simulink model "BD_PAR_SS"  (Simulink 10.3)
settings: Solver=ode1  StartTime=0.0  StopTime=max(cyc_mph(:,1))  FixedStep=1  MaxStep=1  RelTol=1e-3  AbsTol=1e-3
undefined symbols (not defined in the file): acc_elec_eff, acc_elec_pwr, acc_mech_eff, amb_tmp, cs_charge_deplete_bool, cs_electric_decel_spd, cs_electric_launch_spd_hi, cs_electric_launch_spd_lo, cs_hi_soc, cs_lo_soc, cs_off_trq_frac, cyc_avg_time, cyc_cargo_mass, cyc_elevation_init, cyc_filter_bool, cyc_grade, cyc_mph, ess_module_num, ess_on, ess_voc, ex_calc, ex_cat_co_frac, ex_cat_ext_cp, ex_cat_ext_emisv, ex_cat_ext_init_tmp, ex_cat_ext_mass, ex_cat_ext_sarea, ex_cat_hc_frac, ex_cat_i2p_th_cond, ex_cat_i2x_emisv, ex_cat_i2x_th_cond, ex_cat_int_cp, ex_cat_int_init_tmp, ex_cat_int_mass, ex_cat_int_sarea, ex_cat_lim, ex_cat_m2i_th_cond, ex_cat_m2i_tmp, ex_cat_m2p_emisv, ex_cat_mon_cp, ex_cat_mon_init_tmp, ex_cat_mon_mass, ex_cat_mon_sarea, ex_cat_monf_sarea, ex_cat_moni_sarea, ex_cat_nox_frac, ex_cat_p2x_th_cond, ex_cat_pcm_ecp, ex_cat_pcm_mass, ex_cat_pcm_tmp, ex_cat_pipe_cp, ex_cat_pipe_emisv, ex_cat_pipe_init_tmp, ex_cat_pipe_mass, ex_cat_pipe_sarea, ex_cat_pm_frac, ex_cat_tmp_range, ex_gas_cp, ex_manif_cp, ex_manif_emisv ... (+73)
libraries: lib_controls x6, lib_vehicle x3, lib_accessory x2, lib_interactive x1, lib_energy_storage x1, lib_fuel_converter x1
(part 2 of 6)

== system BD_PAR_SS/mechanical accessory loads <acc> ==
  note: from <fc>
  note: from <fc>
  note: torque req
  note: speed req
  note: aux spd req
  note: torque achieved
  note: speed achieved
  note: aux spd achieved
  note: from <fc>
  note: In order to load the engine,
      | the engine must be on and
      | the shaft speed must
      | be greater than zero (fc_spd_est is assumed
      | to bound itself to max fc speed and idle speed)
      |
      | The basic assumption is that the aux. loads
      | will not change the requested engine speed--
      | only the torque
  note: "kill switch" for accessory loads
  In1 : Inport
  In2 : Inport  Port=2
  Constant : Constant  Value=eps
  Demux : Demux  Outputs=2
      settings: DisplayOption=none
  Demux1 : Demux  Outputs=2
      settings: DisplayOption=none
  Logical Operator : Logic
  Mechanical Accessory Loads v2 <acc> : Subsystem  mask{load_on=not(ess_on)*1, acc_max_spd=inf, acc_min_spd=vc_idle_spd*vc_idle_bool+eps, ic_mech_trq=0, ic_mech_pwr=0}
      mask prompts: load_on "Electrical Load Status: 1 on; 0 off"; acc_max_spd "maximum shaft speed for aux. (rad/s)"; acc_min_spd "minimum shaft speed for aux. (rad/s)"; ic_mech_trq "Initial Mechanical Torque of the Accessory Loads (Nm)"; ic_mech_pwr "Initial Mechanical Auxiliary Load Power (W)"
      mask Display: image(imread('bdi_acc_pic.bmp'))
  Mux : Mux  Inputs=3
  Mux1 : Mux  Inputs=3
  Relational Operator : RelationalOperator  Operator=>  RndMeth=Nearest  InputSameDT=on
  Out1 : Outport
  Out2 : Outport  Port=2
  wires:
  [signal_one] -> Mechanical Accessory Loads v2 <acc>/1("requested shaft T and w, out to the driveline  (Nm ; rad/s; rad/s)")
  Mechanical Accessory Loads v2 <acc>/1("requested shaft and belt T and w, in from the prime mover (Nm ; rad/s)") -> Out1/1
  Mechanical Accessory Loads v2 <acc>/2("achieved shaft T and w, out to the driveline (Nm ; rad/s)") -> Out2/1
  [signal_two] -> Mechanical Accessory Loads v2 <acc>/2("achieved shaft and belt T and w, in from the prime mover (Nm ; rad/s)")
  Mux/1 -> [signal_one]
  In1/1 -> Demux/1
  Demux/1 -> Mux/1
  Demux/2 -> Mux/2
  [fc_spd_est] -> Mux/3
  Mux1/1 -> [signal_two]
  In2/1 -> Demux1/1
  Demux1/1 -> Mux1/1
  Demux1/2 -> Mux1/2
  [fc_spd_est] -> Mux1/3
  [engine_on] -> Logical Operator/1
  Logical Operator/1 -> [acc_on]
  [acc_on] -> Mechanical Accessory Loads v2 <acc>/3(accessory on/off)
  [fc_spd_est] -> Relational Operator/1
  Constant/1 -> Relational Operator/2
  Relational Operator/1 -> Logical Operator/2

== system BD_PAR_SS/motor/ controller <mc> par ==
  "torque and speed  req'd at rotor (Nm), (rad/s)" : Inport
  available motor input power (W) : Inport  Port=2
  Block NOTES : Subsystem
      mask Display: disp('Block\nNOTES')
  Constant : Constant  Value=mc_eff_scale
  Demux : Demux  Outputs=2
  Fcn : Fcn  Expr=u[3]-u[1]*u[2]
  Mux2 : Mux  Inputs=2
  Mux3 : Mux  Inputs=3
  N-m drive torque per W input : Subsystem
  Product : Product  SaturateOnIntegerOverflow=on
  Product1 : Product  Inputs=*/  SaturateOnIntegerOverflow=on
  Saturation : Saturate  UpperLimit=max(mc_map_spd)*mc_spd_scale  LowerLimit=0
  Sum : Sum  SaturateOnIntegerOverflow=on
  Sum1 : Sum  Inputs=-+  SaturateOnIntegerOverflow=on
  Switch : Switch  SaturateOnIntegerOverflow=on  InputSameDT=on
  To WS1 : ToWorkspace  VariableName=mc_pwr_loss
      settings: MaxDataPoints=50000
  To WS2 : ToWorkspace  VariableName=mc_tmp
      settings: MaxDataPoints=50000
  To WS4 : ToWorkspace  VariableName=mc_clt_th_pwr
      settings: MaxDataPoints=50000
  To Workspace10 : ToWorkspace  VariableName=mc_ni_trq_out_a  SampleTime=-1
  To Workspace4 : ToWorkspace  VariableName=mc_trq_out_r  SampleTime=-1
  To Workspace5 : ToWorkspace  VariableName=mc_spd_out_r  SampleTime=-1
  To Workspace8 : ToWorkspace  VariableName=mc_pwr_in_a  SampleTime=-1
  To Workspace9 : ToWorkspace  VariableName=mc_pwr_in_r  SampleTime=-1
  do ex calcs? : Constant  Value=mc_th_calc
  documentation10 : Subsystem
      settings: OpenFcn=web(['file:\\\' which('motor_controller.htm')]);
      mask Display: image(imread('doc_man.jpg'))
  effect of inertia (Nm) : Subsystem
  enforce torque limit : Subsystem
  mc tmp : Subsystem  TreatAsAtomicUnit=on
  motor controller logic interface : Subsystem
  motor speed estimator : Subsystem
  motor/controller input power map (W) : Lookup2D  RowIndex=mc_map_spd*mc_spd_scale  ColumnIndex=mc_map_trq*mc_trq_scale  Table=mc_inpwr_map*mc_spd_scale*mc_trq_scale  SaturateOnIntegerOverflow=on  InputSameDT=on
  rotor drive torque available (Nm) : Subsystem
  req'd motor input power (W) : Outport  InitialOutput=0
  "drive torque and speed avail. at rotor (Nm), (rad/s)" : Outport  Port=2  InitialOutput=0
  tag scope: mc_spd_out_a=global, mc_trq_out_a=global
  wires:
  motor/controller input power map (W)/1 -> Product/1, Switch/2, Product1/1
  Product/1 -> Switch/3
  Product1/1 -> Switch/1
  Switch/1 -> N-m drive torque per W input/1(req'd input power (W)), motor controller logic interface/2(P_mc_in_1lim)
  Constant/1 -> Product/2, Product1/2
  motor speed estimator/1(Out1) -> motor/controller input power map (W)/1, enforce torque limit/2(limited motor speed (rad/s))
  Saturation/1 -> effect of inertia (Nm)/1(mc_spd_out_a), motor speed estimator/1(mc_spd_out_a), Mux3/2, Mux2/2, [mc_spd_out_a]
  Sum1/1 -> Mux3/1, Mux2/1, [mc_trq_out_a]
  N-m drive torque per W input/1(Nm per W) -> rotor drive torque available (Nm)/1(torque per unit input power (N-m/W))
  Sum/1 -> enforce torque limit/1(req'd motor torque (Nm))
  effect of inertia (Nm)/1(out_1) -> Sum/2, Sum1/1
  enforce torque limit/1(limited motor torque (Nm)) -> N-m drive torque per W input/2(req'd rotor drive torque (Nm)), motor/controller input power map (W)/2
  motor controller logic interface/1(P_mc_in_r) -> To Workspace9/1, req'd motor input power (W)/1
  Mux2/1 -> "drive torque and speed avail. at rotor (Nm), (rad/s)"/1
  Mux3/1 -> Fcn/1
  Fcn/1 -> To WS1/1, mc tmp/1(Qmc_gen)
  do ex calcs?/1 -> mc tmp/Enable
  mc tmp/1(Tmc) -> To WS2/1
  mc tmp/2(Qmc_clt) -> To WS4/1
  [v_prev] -> mc tmp/2(veh spd)
  [key_on] -> mc tmp/3(key ON?)
  Demux/2 -> Saturation/1, To Workspace5/1, motor controller logic interface/1(w_mc_out_r)
  available motor input power (W)/1 -> Mux3/3, To Workspace8/1, rotor drive torque available (Nm)/2(available input power (W))
  Demux/1 -> Sum/1, To Workspace4/1
  "torque and speed  req'd at rotor (Nm), (rad/s)"/1 -> Demux/1
  rotor drive torque available (Nm)/1(rotor drive torque available) -> Sum1/2, To Workspace10/1

== system BD_PAR_SS/par <cs> config ==
  "trq and spd req'd into clutch (N*m, rad/s)" : Inport
  electric assist control strategy <cs> : lib_controls/electric assist control strategy <cs>  SystemSampleTime=-1  VariantActivationTime=update diagram  Latency=0  AutoFrameSizeCalculation=off
  "trq and spd req'd from engine (N*m, rad/s)" : Outport
  wires:
  "trq and spd req'd into clutch (N*m, rad/s)"/1 -> electric assist control strategy <cs>/1
  electric assist control strategy <cs>/1 -> "trq and spd req'd from engine (N*m, rad/s)"/1

== system BD_PAR_SS/power bus <pb> ==
  req'd power output (W) : Inport
  power available from generator (W) : Inport  Port=2
  power available from energy storage (W) : Inport  Port=3
  Abs : Abs  SaturateOnIntegerOverflow=on
  Abs1 : Abs  SaturateOnIntegerOverflow=on
  Block NOTES : Subsystem
      mask Display: disp('Block\nNOTES')
  Constant : Constant  Value=1e-9
  Constant1 : Constant  Value=1e-11
  Constant2 : Constant  Value=0
  Constant7 : Constant  Value=ess_on
  Constant8 : Constant  Value=0
  Relational Operator : RelationalOperator  Operator=<=  RndMeth=Nearest  InputSameDT=on
  Relational Operator1 : RelationalOperator  Operator=<=  RndMeth=Nearest  InputSameDT=on
  Sum1 : Sum  Inputs=+-  SaturateOnIntegerOverflow=on
  Sum2 : Sum  SaturateOnIntegerOverflow=on
  Switch : Switch  Threshold=eps  SaturateOnIntegerOverflow=on  InputSameDT=on
  Switch1 : Switch  Threshold=eps  SaturateOnIntegerOverflow=on  InputSameDT=on
  To Workspace8 : ToWorkspace  VariableName=pb_pwr_out_a  SampleTime=-1
  To Workspace9 : ToWorkspace  VariableName=pb_pwr_out_r  SampleTime=-1
  not(and(u1,u2)) : Logic  Operator=NAND
  power req'd from generator (W) : Outport
  power req'd from energy storage (W) : Outport  Port=2
  output power  available at bus : Outport  Port=3
  wires:
  power available from energy storage (W)/1 -> Sum2/2
  Constant8/1 -> Switch1/3
  Constant7/1 -> Switch1/2
  Switch1/1 -> power req'd from energy storage (W)/1
  Sum1/1 -> Switch1/1
  Constant/1 -> Relational Operator/2
  Abs/1 -> Relational Operator/1
  Sum2/1 -> Switch/1, Abs/1
  Switch/1 -> output power  available at bus/1, To Workspace8/1
  Constant1/1 -> Relational Operator1/2
  Abs1/1 -> Relational Operator1/1
  Relational Operator1/1 -> not(and(u1,u2))/2
  not(and(u1,u2))/1 -> Switch/2
  Constant2/1 -> Switch/3
  Relational Operator/1 -> not(and(u1,u2))/1
  power available from generator (W)/1 -> Sum1/2, Sum2/1
  req'd power output (W)/1 -> power req'd from generator (W)/1, Sum1/1, To Workspace9/1, Abs1/1

== system BD_PAR_SS/torque coupler <tc> ==
  "torque and speed req'd at output side of torque coupler (Nm), (rad/s)" : Inport
  "torque and speed avail. at main input (Nm), (rad/s)" : Inport  Port=2
  "torque and speed avail. at motor input to tc (Nm), (rad/s)" : Inport  Port=3
  Block NOTES : Subsystem
      mask Display: disp('Block\nNOTES')
  Demux : Demux  Outputs=2
  Demux1 : Demux  Outputs=2
  Demux2 : Demux  Outputs=2
  MinMax : MinMax  Inputs=2
  MinMax1 : MinMax  Inputs=2
  Mux : Mux  Inputs=2
  Mux1 : Mux  Inputs=2
  Mux2 : Mux  Inputs=2
  Product : Product  Inputs=1  SaturateOnIntegerOverflow=on
  Product1 : Product  Inputs=1  SaturateOnIntegerOverflow=on
  To Workspace2 : ToWorkspace  VariableName=tc_trq_out_r  SampleTime=-1
  To Workspace3 : ToWorkspace  VariableName=tc_spd_out_r  SampleTime=-1
  To Workspace4 : ToWorkspace  VariableName=tc_trq_out_a  SampleTime=-1
  To Workspace5 : ToWorkspace  VariableName=tc_spd_out_a  SampleTime=-1
  To Workspace6 : ToWorkspace  VariableName=tc_pwr_in_a  SampleTime=-1
  effect of motor torque at output of tc (Nm) : Gain  Gain=tc_mc_to_fc_ratio  SaturateOnIntegerOverflow=on
  help : Subsystem
      settings: OpenFcn=web(['file:\\\' which('torque_coupler.htm')]);
      mask Display: image(imread('doc_man.jpg'))
  loss (Nm) : Subsystem
  speed of output gear corresponding to motor spd (rad/s) : Gain  Gain=1/tc_mc_to_fc_ratio  SaturateOnIntegerOverflow=on
  speed req'd of motor (rad/s) : Gain  Gain=tc_mc_to_fc_ratio  SaturateOnIntegerOverflow=on
  "sum " : Sum  SaturateOnIntegerOverflow=on
  torque avail. at output side of tc (Nm) : Sum  Inputs=-++  SaturateOnIntegerOverflow=on
  total torque req'd at output gear (Nm) : Sum  SaturateOnIntegerOverflow=on
  total torque req'd of motor (Nm) : Gain  Gain=1/tc_mc_to_fc_ratio  SaturateOnIntegerOverflow=on
  unmet torque request (Nm) : Sum  Inputs=+-  SaturateOnIntegerOverflow=on
  "torque and speed req'd at main input to torque coupler (Nm), (rad/s)" : Outport  InitialOutput=0
  "torque and speed req'd at motor input to torque coupler (Nm), (rad/s)" : Outport  Port=2  InitialOutput=0
  "torque and speed avail. at output side of torque coupler (Nm), (rad/s)" : Outport  Port=3  InitialOutput=0
  wires:
  Product1/1 -> "sum "/2
  "torque and speed avail. at motor input to tc (Nm), (rad/s)"/1 -> Product1/1, Demux2/1
  "torque and speed avail. at main input (Nm), (rad/s)"/1 -> Product/1, Demux1/1
  Product/1 -> "sum "/1
  "sum "/1 -> To Workspace6/1
  Mux/1 -> "torque and speed req'd at main input to torque coupler (Nm), (rad/s)"/1
  "torque and speed req'd at output side of torque coupler (Nm), (rad/s)"/1 -> Demux/1
  Demux/2 -> loss (Nm)/1(tc output speed (rad/s)), Mux/2, MinMax/1, To Workspace3/1
  total torque req'd at output gear (Nm)/1 -> Mux/1, unmet torque request (Nm)/1
  unmet torque request (Nm)/1 -> total torque req'd of motor (Nm)/1
  Demux1/2 -> MinMax/2
  Mux1/1 -> "torque and speed req'd at motor input to torque coupler (Nm), (rad/s)"/1
  total torque req'd of motor (Nm)/1 -> Mux1/1
  speed req'd of motor (rad/s)/1 -> Mux1/2
  loss (Nm)/1(drag torque (Nm)) -> total torque req'd at output gear (Nm)/2, torque avail. at output side of tc (Nm)/1
  Demux1/1 -> unmet torque request (Nm)/2, torque avail. at output side of tc (Nm)/2
  Demux2/1 -> effect of motor torque at output of tc (Nm)/1
  effect of motor torque at output of tc (Nm)/1 -> torque avail. at output side of tc (Nm)/3
  Mux2/1 -> "torque and speed avail. at output side of torque coupler (Nm), (rad/s)"/1
  Demux2/2 -> speed of output gear corresponding to motor spd (rad/s)/1
  speed of output gear corresponding to motor spd (rad/s)/1 -> MinMax1/2
  MinMax/1 -> speed req'd of motor (rad/s)/1, MinMax1/1
  Demux/1 -> total torque req'd at output gear (Nm)/1, To Workspace2/1
  torque avail. at output side of tc (Nm)/1 -> Mux2/1, To Workspace4/1
  MinMax1/1 -> Mux2/2, To Workspace5/1

== system BD_PAR_SS/vehicle <veh> ==
  vehicle speed req'd at end of time step (m/s) : Inport
  tractive force and linear speed achievable (N) : Inport  Port=2
  "(m/s) -> (mph)1" : Gain  Gain=2.23713646532438  SaturateOnIntegerOverflow=on
  Block NOTES : Subsystem
      mask Display: disp('Block\nNOTES')
  Demux1 : Demux  Outputs=2
  Gain : Gain  Gain=0.5  SaturateOnIntegerOverflow=on
  Memory : Memory  InitialCondition=cyc_mph(1,2)*.447
  Mux : Mux  Inputs=2
  Rolling Resistance Force (N) : ToWorkspace  VariableName=Fr  SampleTime=-1
  Sum : Sum  SaturateOnIntegerOverflow=on
  Sum1 : Sum  Inputs=++++  SaturateOnIntegerOverflow=on
  To Workspace2 : ToWorkspace  VariableName=veh_force_r  SampleTime=-1
  To Workspace3 : ToWorkspace  VariableName=veh_spd_r  SampleTime=-1
  To Workspace4 : ToWorkspace  VariableName=veh_force_a  SampleTime=-1
  To Workspace5 : ToWorkspace  VariableName=veh_spd_a  SampleTime=-1
  force req'd to accelerate (N) : Subsystem
  force req'd to ascend (N) : Subsystem
  force req'd to overcome aerodynamic drag (N) : Subsystem
  help : Subsystem
      settings: OpenFcn=web(['file:\\\' which('vehicle.htm')]);
      mask Display: image(imread('doc_man.jpg'))
  record achieved force outputs : Subsystem
  rolling resistance force : Subsystem  BlockChoice=force req'd to overcome rolling resistance (N)
      settings: AttributesFormatString=%<BlockChoice>  TemplateBlock=lib_vehicle/Submodels/rolling resistance force  MemberBlocks=force req'd to overcome rolling resistance (N),force req'd to overcome rolling resistance (N) j2452
  vehicle speed : Subsystem  BlockChoice=vehicle speed (m/s)
      settings: AttributesFormatString=%<BlockChoice>  TemplateBlock=lib_vehicle/Submodels/vehicle speed  MemberBlocks=vehicle speed (m/s),vehicle speed (m/s) j2452
  "tractive force and speed required of tire and wheel (N), (m/s)" : Outport  InitialOutput=0
  tag scope: mpha=global, v_prev=global
  wires:
  vehicle speed/1(vehicle speed achievable at end of time step (m/s)) -> record achieved force outputs/2(spd), "(m/s) -> (mph)1"/1, Memory/1
  tractive force and linear speed achievable (N)/1 -> vehicle speed/2("available tractive force and linear speed (N), (m/s)"), Demux1/1
  Gain/1 -> rolling resistance force/1(average vehicle speed over time step (m/s)), force req'd to overcome aerodynamic drag (N)/1(average vehicle speed over time step (m/s)), Mux/2, To Workspace3/1, force req'd to ascend (N)/1(average vehicle speed over time step (m/s))
  Sum/1 -> Gain/1
  vehicle speed req'd at end of time step (m/s)/1 -> force req'd to accelerate (N)/1(v(m/s)), Sum/1
  Mux/1 -> "tractive force and speed required of tire and wheel (N), (m/s)"/1
  Sum1/1 -> Mux/1, To Workspace2/1
  Demux1/1 -> To Workspace4/1
  Demux1/2 -> To Workspace5/1
  force req'd to overcome aerodynamic drag (N)/1(D aero(N)) -> Sum1/3
  force req'd to accelerate (N)/1((N)) -> Sum1/4
  Memory/1 -> record achieved force outputs/1(spd_prev), [v_prev], vehicle speed/1(vehicle speed at beginning of time step (m/s)), force req'd to accelerate (N)/2(v prev), Sum/2
  "(m/s) -> (mph)1"/1 -> [mpha]
  force req'd to ascend (N)/1((N)) -> Sum1/2
  rolling resistance force/1(Fr (N)) -> Rolling Resistance Force (N)/1, Sum1/1

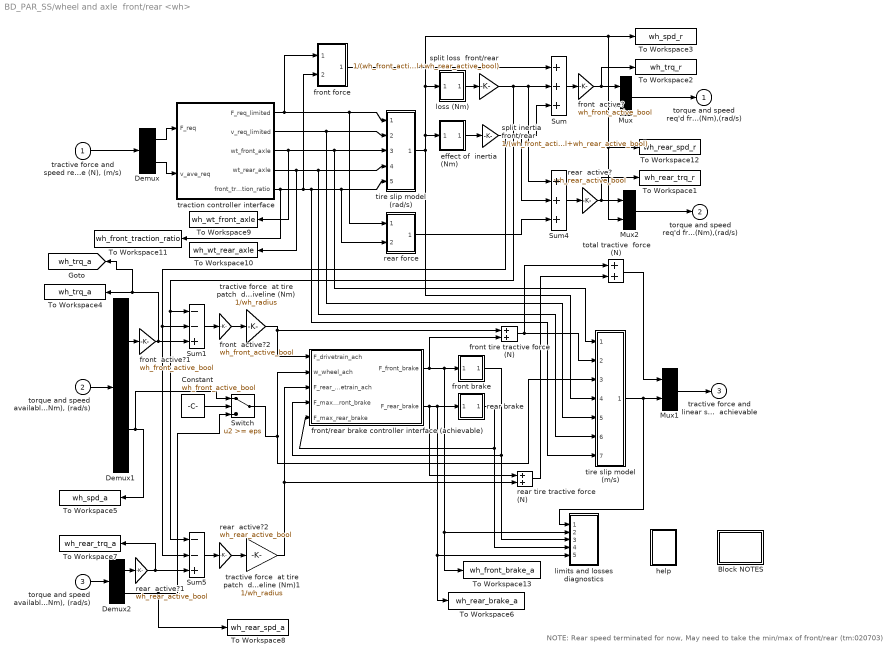
== system BD_PAR_SS/wheel and axle  front/rear <wh> ==
  note: NOTE: Rear speed terminated for now, May need to take the min/max of front/rear (tm:020703)
  "tractive force and speed req'd of tire/road interface (N), (m/s)" : Inport
  "torque and speed available from drivetrain into front axle (Nm), (rad/s)" : Inport  Port=2
  "torque and speed available from drivetrain into rear axle (Nm), (rad/s)" : Inport  Port=3
  Block NOTES : Subsystem
      mask Display: disp('Block\nNOTES')
  Constant : Constant  Value=wh_front_active_bool
  Demux : Demux  Outputs=2
  Demux1 : Demux  Outputs=2
  Demux2 : Demux  Outputs=2
  Mux : Mux  Inputs=2
  Mux1 : Mux  Inputs=2
  Mux2 : Mux  Inputs=2
  Sum : Sum  Inputs=+++  SaturateOnIntegerOverflow=on
  Sum1 : Sum  Inputs=--+  SaturateOnIntegerOverflow=on
  Sum4 : Sum  Inputs=+++  SaturateOnIntegerOverflow=on
  Sum5 : Sum  Inputs=--+  SaturateOnIntegerOverflow=on
  Switch : Switch  Threshold=eps  SaturateOnIntegerOverflow=on  InputSameDT=on
  To Workspace1 : ToWorkspace  VariableName=wh_rear_trq_r  SampleTime=-1
  To Workspace10 : ToWorkspace  VariableName=wh_wt_rear_axle  SampleTime=-1
  To Workspace11 : ToWorkspace  VariableName=wh_front_traction_ratio  SampleTime=-1
  To Workspace12 : ToWorkspace  VariableName=wh_rear_spd_r  SampleTime=-1
  To Workspace13 : ToWorkspace  VariableName=wh_front_brake_a  SampleTime=-1
  To Workspace2 : ToWorkspace  VariableName=wh_trq_r  SampleTime=-1
  To Workspace3 : ToWorkspace  VariableName=wh_spd_r  SampleTime=-1
  To Workspace4 : ToWorkspace  VariableName=wh_trq_a  SampleTime=-1
  To Workspace5 : ToWorkspace  VariableName=wh_spd_a  SampleTime=-1
  To Workspace6 : ToWorkspace  VariableName=wh_rear_brake_a  SampleTime=-1
  To Workspace7 : ToWorkspace  VariableName=wh_rear_trq_a  SampleTime=-1
  To Workspace8 : ToWorkspace  VariableName=wh_rear_spd_a  SampleTime=-1
  To Workspace9 : ToWorkspace  VariableName=wh_wt_front_axle  SampleTime=-1
  effect of  inertia (Nm) : Subsystem
  front  active? : Gain  Gain=wh_front_active_bool  SaturateOnIntegerOverflow=on
  front  active?1 : Gain  Gain=wh_front_active_bool  SaturateOnIntegerOverflow=on
  front  active?2 : Gain  Gain=wh_front_active_bool  SaturateOnIntegerOverflow=on
  front brake : Subsystem
  front force : Subsystem
  front tire tractive force (N) : Sum  SaturateOnIntegerOverflow=on
  front/rear brake controller interface (achievable) : Subsystem
  help : Subsystem
      settings: OpenFcn=web(['file:\\\' which('advisor_doc.htm')]);
      mask Display: image(imread('doc_man.jpg'))
  limits and losses diagnostics : Subsystem
  loss (Nm) : Subsystem
  rear  active? : Gain  Gain=wh_rear_active_bool  SaturateOnIntegerOverflow=on
  rear  active?1 : Gain  Gain=wh_rear_active_bool  SaturateOnIntegerOverflow=on
  rear  active?2 : Gain  Gain=wh_rear_active_bool  SaturateOnIntegerOverflow=on
  rear brake : Subsystem
  rear force : Subsystem
  rear tire tractive force (N) : Sum  SaturateOnIntegerOverflow=on
  split inertia front/rear : Gain  Gain=1/(wh_front_active_bool+wh_rear_active_bool)  SaturateOnIntegerOverflow=on
  split loss  front/rear : Gain  Gain=1/(wh_front_active_bool+wh_rear_active_bool)  SaturateOnIntegerOverflow=on
  tire slip model (m/s) : Subsystem
  tire slip model (rad/s) : Subsystem
  total tractive  force (N) : Sum  SaturateOnIntegerOverflow=on
  traction controller interface : Subsystem
  tractive force  at tire patch  due to driveline (Nm) : Gain  Gain=1/wh_radius  SaturateOnIntegerOverflow=on
  tractive force  at tire patch  due to driveline (Nm)1 : Gain  Gain=1/wh_radius  SaturateOnIntegerOverflow=on
  torque and speed req'd from drivetrain into front axle (Nm),(rad/s) : Outport  InitialOutput=0
  torque and speed req'd from drivetrain into rear axle (Nm),(rad/s) : Outport  Port=2  InitialOutput=0
  tractive force and linear speed  achievable : Outport  Port=3  InitialOutput=0
  tag scope: wh_trq_a=global
  wires:
  Demux1/2 -> To Workspace5/1, Switch/1
  Constant/1 -> Switch/2
  front  active?2/1 -> tractive force  at tire patch  due to driveline (Nm)/1
  rear  active?2/1 -> tractive force  at tire patch  due to driveline (Nm)1/1
  rear  active?1/1 -> Sum5/3, To Workspace7/1
  front  active?1/1 -> Sum1/3, [wh_trq_a], To Workspace4/1
  rear  active?/1 -> Mux2/1, To Workspace1/1
  front  active?/1 -> To Workspace2/1, Mux/1
  Demux2/2 -> Switch/3, To Workspace8/1
  Demux2/1 -> rear  active?1/1
  rear tire tractive force (N)/1 -> total tractive  force (N)/2
  tractive force  at tire patch  due to driveline (Nm)1/1 -> rear tire tractive force (N)/2, front/rear brake controller interface (achievable)/3(F_rear_drivetrain_ach)
  "torque and speed available from drivetrain into rear axle (Nm), (rad/s)"/1 -> Demux2/1
  Sum5/1 -> rear  active?2/1
  traction controller interface/4(wt_rear_axle) -> To Workspace10/1, tire slip model (m/s)/6(weight borne by  rear axle (N)), tire slip model (rad/s)/4(weight borne by  rear axle (N)1)
  split inertia front/rear/1 -> Sum5/2, Sum1/2, Sum4/2, Sum/3
  split loss  front/rear/1 -> Sum5/1, Sum1/1, Sum4/1, Sum/2
  Mux2/1 -> torque and speed req'd from drivetrain into rear axle (Nm),(rad/s)/1
  Sum4/1 -> rear  active?/1
  rear force/1(Out1) -> Sum4/3
  traction controller interface/5(front_traction_ratio) -> To Workspace11/1, front force/2(In2), rear force/2(In2), tire slip model (rad/s)/5(front traction ratio), tire slip model (m/s)/7(front fraction)
  Demux/1 -> traction controller interface/1(F_req)
  front/rear brake controller interface (achievable)/2(F_rear_brake) -> To Workspace6/1, limits and losses diagnostics/5(rear brake), rear brake/1(F_brake), rear tire tractive force (N)/1
  traction controller interface/1(F_req_limited) -> front force/1(In1), tire slip model (rad/s)/1(total tractive  force requested (N)), rear force/1(In1)
  Switch/1 -> tire slip model (m/s)/3(axle speed available (rad/s)), front/rear brake controller interface (achievable)/2(w_wheel_ach)
  Demux1/1 -> front  active?1/1
  Sum/1 -> front  active?/1
  Mux/1 -> torque and speed req'd from drivetrain into front axle (Nm),(rad/s)/1
  traction controller interface/3(wt_front_axle) -> To Workspace9/1, tire slip model (m/s)/1(weight borne  by front axle (N)), tire slip model (rad/s)/3(weight borne by front axle (N))
  rear brake/1(F_brake_max) -> limits and losses diagnostics/4(rear brake max), front/rear brake controller interface (achievable)/5(F_max_rear_brake)
  front brake/1(F_brake_max) -> limits and losses diagnostics/3(front brake max), front/rear brake controller interface (achievable)/4(F_max_front_brake)
  front tire tractive force (N)/1 -> total tractive  force (N)/1, tire slip model (m/s)/2(total tractive  force available (N))
  front/rear brake controller interface (achievable)/1(F_front_brake) -> To Workspace13/1, limits and losses diagnostics/2(front brake), front brake/1(F_brake), front tire tractive force (N)/2
  "torque and speed available from drivetrain into front axle (Nm), (rad/s)"/1 -> Demux1/1
  total tractive  force (N)/1 -> Mux1/1
  Mux1/1 -> tractive force and linear speed  achievable/1
  front force/1(Out1) -> Sum/1
  tire slip model (rad/s)/1(slip-augmented rotational speed (rad/s)) -> tire slip model (m/s)/4(axle speed req'd (rad/s)), To Workspace12/1, Mux2/2, Mux/2, To Workspace3/1, loss (Nm)/1(axle speed (rad/s)), effect of  inertia (Nm)/1(axle input speed (rad/s))
  "tractive force and speed req'd of tire/road interface (N), (m/s)"/1 -> Demux/1
  loss (Nm)/1(drag torque (Nm)) -> split loss  front/rear/1
  effect of  inertia (Nm)/1(inertia torque (Nm)) -> split inertia front/rear/1
  Sum1/1 -> front  active?2/1
  tractive force  at tire patch  due to driveline (Nm)/1 -> front tire tractive force (N)/1, front/rear brake controller interface (achievable)/1(F_drivetrain_ach)
  tire slip model (m/s)/1(possible vehicle speed (m/s)) -> limits and losses diagnostics/1(speed), Mux1/2
  Demux/2 -> traction controller interface/2(v_ave_req)
  traction controller interface/2(v_req_limited) -> tire slip model (m/s)/5(vehicle speed required (m/s)), tire slip model (rad/s)/2(requested time-step average vehicle speed (m/s))

== system BD_PAR_SS/<vc> par/config traction control ==
  time-average vehicle speed  req'd (m/s) : Inport
  vehicle speed at beginning of time  step (m/s) : Inport  Port=2
  total tractive force req'd (N) : Inport  Port=3
  traction control 2 axle : lib_controls/SubSystem/traction control 2 axle  SystemSampleTime=-1  VariantActivationTime=update diagram  Latency=0  AutoFrameSizeCalculation=off
  req'd force (N) : Outport
  req'd speed (m/s) : Outport  Port=2
  weight on front axle (N) : Outport  Port=3
  weight on rear axle (N) : Outport  Port=4
  front/total  traction ratio : Outport  Port=5
  wires:
  time-average vehicle speed  req'd (m/s)/1 -> traction control 2 axle/1
  vehicle speed at beginning of time  step (m/s)/1 -> traction control 2 axle/2
  total tractive force req'd (N)/1 -> traction control 2 axle/3
  traction control 2 axle/1 -> req'd force (N)/1
  traction control 2 axle/2 -> req'd speed (m/s)/1
  traction control 2 axle/3 -> weight on front axle (N)/1
  traction control 2 axle/4 -> weight on rear axle (N)/1
  traction control 2 axle/5 -> front/total  traction ratio/1

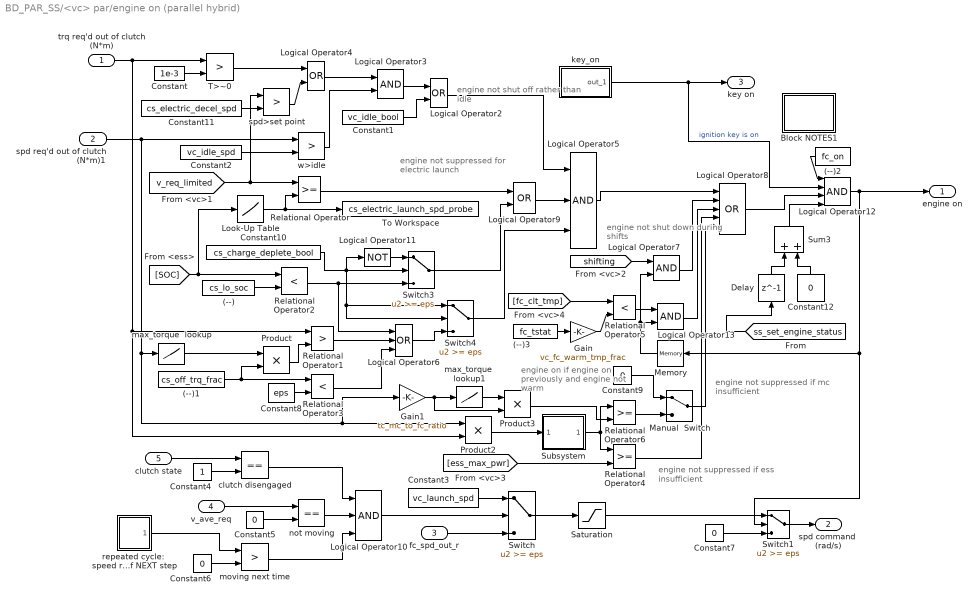
== system BD_PAR_SS/<vc> par/engine on (parallel hybrid) ==
  note: engine not suppressed
      | if mc insufficient
  note: engine not shut
      | down during shifts
  note: engine on if engine on
      | previously and engine
      | not warm
  note: engine not shut off
      |  rather than idle
  note: engine not
      | suppressed for
      | electric launch
  note: engine not suppressed if
      | ess insufficient
  trq req'd out of clutch (N*m) : Inport
  spd req'd out of clutch (N*m)1 : Inport  Port=2
  fc_spd_out_r : Inport  Port=3
  v_ave_req : Inport  Port=4
  clutch state : Inport  Port=5
  (--) : Constant  Value=cs_lo_soc
  (--)1 : Constant  Value=cs_off_trq_frac
  (--)2 : Constant  Value=fc_on
  (--)3 : Constant  Value=fc_tstat
  Block NOTES1 : Subsystem
      mask Display: disp('Block\nNOTES')
  Constant : Constant  Value=1e-3
  Constant1 : Constant  Value=vc_idle_bool
  Constant10 : Constant  Value=cs_charge_deplete_bool
  Constant11 : Constant  Value=cs_electric_decel_spd
  Constant{5..7,9,12} (5 alike) : Constant  Value=0
  Constant2 : Constant  Value=vc_idle_spd
  Constant3 : Constant  Value=vc_launch_spd
  Constant4 : Constant
  Constant8 : Constant  Value=eps
  Delay : Delay  DelayLength=1  InitialCondition=1
  Gain : Gain  Gain=vc_fc_warm_tmp_frac  SaturateOnIntegerOverflow=on  OutDataTypeStr=Inherit: Same as input  ParamDataTypeStr=Inherit: Same as input
  Gain1 : Gain  Gain=tc_mc_to_fc_ratio  SaturateOnIntegerOverflow=on  OutDataTypeStr=Inherit: Same as input  ParamDataTypeStr=Inherit: Same as input
  Logical Operator10 : Logic  Inputs=3
  Logical Operator11 : Logic  Operator=NOT  Inputs=1
  Logical Operator12 : Logic  Inputs=4
  Logical Operator13 : Logic
  Logical Operator2 : Logic  Operator=OR
  Logical Operator3 : Logic
  Logical Operator4 : Logic  Operator=OR
  Logical Operator5 : Logic  Inputs=3
  Logical Operator6 : Logic  Operator=OR  Inputs=3
  Logical Operator7 : Logic
  Logical Operator8 : Logic  Operator=OR  Inputs=5
  Logical Operator9 : Logic  Operator=OR
  Look-Up Table : Lookup  InputValues=[cs_lo_soc cs_hi_soc cs_hi_soc+eps]  Table=[cs_electric_launch_spd_lo cs_electric_launch_spd_hi cs_electric_launch_spd_hi]  SaturateOnIntegerOverflow=on
  Manual  Switch : ManualSwitch
  Memory : Memory  InitialCondition=cyc_mph(1,2)>0
  Product : Product  InputSameDT=on  RndMeth=Zero  SaturateOnIntegerOverflow=on  OutDataTypeStr=Inherit: Same as first input
  Product2 : Product  InputSameDT=on  RndMeth=Zero  SaturateOnIntegerOverflow=on  OutDataTypeStr=Inherit: Same as first input
  Product3 : Product  InputSameDT=on  RndMeth=Zero  SaturateOnIntegerOverflow=on  OutDataTypeStr=Inherit: Same as first input
  Relational Operator : RelationalOperator  RndMeth=Nearest  InputSameDT=on
  Relational Operator1 : RelationalOperator  Operator=>  RndMeth=Nearest  InputSameDT=on
  Relational Operator2 : RelationalOperator  Operator=<  RndMeth=Nearest  InputSameDT=on
  Relational Operator3 : RelationalOperator  Operator=<  RndMeth=Nearest  InputSameDT=on
  Relational Operator4 : RelationalOperator  RndMeth=Nearest  InputSameDT=on
  Relational Operator5 : RelationalOperator  Operator=<  RndMeth=Nearest  InputSameDT=on
  Relational Operator6 : RelationalOperator  RndMeth=Nearest  InputSameDT=on
  Saturation : Saturate  UpperLimit=max(fc_map_spd)*fc_spd_scale  LowerLimit=vc_idle_spd*vc_idle_bool
  Subsystem : Subsystem  mask(Running Average){n=3}
      mask prompts: n "Averaging Time Steps (#)"
      mask help: Running Average
      mask Help: Output is the average of the last (Averaging Time) seconds of input.
      mask Display: disp('Running\nAverage')
  Sum3 : Sum  Inputs=+|+
  Switch{,1,3..4} (4 alike) : Switch  Threshold=eps  SaturateOnIntegerOverflow=on  InputSameDT=on
  T>~0 : RelationalOperator  Operator=>  RndMeth=Nearest  InputSameDT=on
  To Workspace : ToWorkspace  VariableName=cs_electric_launch_spd_probe  SampleTime=-1
  clutch disengaged : RelationalOperator  Operator===  RndMeth=Nearest  InputSameDT=on
  key_on : Subsystem  mask(Repeating table){t=vc_key_on(:,1), y=vc_key_on(:,2)}
      mask prompts: t "Time values:"; y "Output values:"
      mask help:
      | Repeating table.
      | Enter values of time and output for first cycle.
      mask init:
      | period = max(t);
      mask Help: Repeats cycle given in table. Time values should be monotonically increasing.
  max_torque  lookup : Lookup  InputValues=fc_map_spd*fc_spd_scale  Table=fc_max_trq*fc_trq_scale  SaturateOnIntegerOverflow=on
  max_torque  lookup1 : Lookup  InputValues=mc_map_spd*mc_spd_scale  Table=mc_max_trq*mc_trq_scale*mc_overtrq_factor  SaturateOnIntegerOverflow=on
  moving next time : RelationalOperator  Operator=>  RndMeth=Nearest  InputSameDT=on
  not moving : RelationalOperator  Operator===  RndMeth=Nearest  InputSameDT=on
  repeated cycle:  speed required at end of NEXT step : Subsystem  mask(Forward looking repeating table){t=cyc_mph(:,1), y=cyc_mph(:,2)}
      mask prompts: t "Time values:"; y "Output values:"
      mask help:
      | Forward looking repeating table.
      | Enter values of time and output for first cycle.
      mask init:
      | period = max(t);
      mask Help: Repeats cycle given in table with a one time step forward offset. Time values should be monotonically increasing.
  spd>set point : RelationalOperator  Operator=>  RndMeth=Nearest  InputSameDT=on
  w>idle : RelationalOperator  Operator=>  RndMeth=Nearest  InputSameDT=on
  engine on : Outport
  spd command  (rad/s) : Outport  Port=2
  key on : Outport  Port=3
  wires:
  Subsystem/1(out_1) -> Relational Operator6/1, Relational Operator4/1
  Product3/1 -> Relational Operator6/2
  [ess_max_pwr] -> Relational Operator4/2
  [v_req_limited] -> spd>set point/1, Relational Operator/1
  T>~0/1 -> Logical Operator4/1
  Logical Operator4/1 -> Logical Operator3/1
  spd>set point/1 -> Logical Operator4/2
  Constant11/1 -> spd>set point/2
  spd req'd out of clutch (N*m)1/1 -> w>idle/1, Gain1/1, Product2/1, max_torque  lookup/1
  w>idle/1 -> Logical Operator3/2
  Constant2/1 -> w>idle/2
  Constant9/1 -> Manual  Switch/1
  Manual  Switch/1 -> Logical Operator8/5
  Relational Operator6/1 -> Manual  Switch/2
  Gain1/1 -> Product3/2, max_torque  lookup1/1
  max_torque  lookup1/1 -> Product3/1
  Relational Operator3/1 -> Logical Operator6/3
  Product2/1 -> Subsystem/1(in_1)
  Constant4/1 -> clutch disengaged/2
  clutch state/1 -> clutch disengaged/1
  Constant5/1 -> not moving/2
  v_ave_req/1 -> not moving/1
  not moving/1 -> Logical Operator10/2
  moving next time/1 -> Logical Operator10/3
  clutch disengaged/1 -> Logical Operator10/1
  Constant6/1 -> moving next time/2
  repeated cycle:  speed required at end of NEXT step/1(out_1) -> moving next time/1
  Constant7/1 -> Switch1/3
  Switch1/1 -> spd command  (rad/s)/1
  Saturation/1 -> Switch1/1
  fc_spd_out_r/1 -> Switch/3
  Logical Operator10/1 -> Switch/2
  Switch/1 -> Saturation/1
  Constant3/1 -> Switch/1
  Relational Operator4/1 -> Logical Operator8/4
  (--)/1 -> Relational Operator2/2
  [SOC] -> Look-Up Table/1, Relational Operator2/1
  Logical Operator11/1 -> Switch3/1
  Relational Operator2/1 -> Logical Operator6/1, Switch3/3
  Constant10/1 -> Logical Operator11/1, Switch3/2, Switch4/2, Switch4/1
  Look-Up Table/1 -> To Workspace/1, Relational Operator/2
  Relational Operator/1 -> Logical Operator9/1
  Switch4/1 -> Logical Operator5/3
  Logical Operator9/1 -> Logical Operator5/2
  Logical Operator2/1 -> Logical Operator5/1
  key_on/1(out_1) -> Logical Operator12/2, key on/1  "ignition key is on"
  Logical Operator8/1 -> Logical Operator12/3
  (--)3/1 -> Gain/1
  Gain/1 -> Relational Operator5/2
  Logical Operator13/1 -> Logical Operator8/3
  [fc_clt_tmp] -> Relational Operator5/1
  Relational Operator5/1 -> Logical Operator13/1
  Memory/1 -> Logical Operator13/2, Logical Operator7/2
  Relational Operator1/1 -> Logical Operator6/2
  Logical Operator5/1 -> Logical Operator8/1
  Logical Operator3/1 -> Logical Operator2/1
  Constant1/1 -> Logical Operator2/2
  trq req'd out of clutch (N*m)/1 -> Relational Operator1/1, Product2/2, T>~0/1
  Logical Operator7/1 -> Logical Operator8/2
  [shifting] -> Logical Operator7/1
  Constant/1 -> T>~0/2
  Switch3/1 -> Logical Operator9/2
  Logical Operator6/1 -> Switch4/3
  Constant8/1 -> Relational Operator3/2
  (--)1/1 -> Relational Operator3/1, Product/2
  Product/1 -> Relational Operator1/2
  max_torque  lookup/1 -> Product/1
  (--)2/1 -> Logical Operator12/1
  Logical Operator12/1 -> engine on/1, Memory/1, Switch1/2
  [ss_set_engine_status] -> Delay/1
  Constant12/1 -> Sum3/2
  Sum3/1 -> Logical Operator12/4
  Delay/1 -> Sum3/1

== system BD_PAR_SS/<vc> par/motor controller logic ==
  bus voltage : Inport
  req'd input power (W) : Inport  Port=2
  req'd output spd (rad/s) : Inport  Port=3
  shifting : Inport  Port=4
  Abs : Abs  SaturateOnIntegerOverflow=on
  Abs1 : Abs  SaturateOnIntegerOverflow=on
  Block NOTES : Subsystem
      mask Display: disp('Block\nNOTES')
  Constant : Constant  Value=mc_max_crrnt
  Constant1 : Constant  Value=0.001
  Constant2 : Constant  Value=0
  Logical Operator1 : Logic  Operator=NOT  Inputs=1
  Memory : Memory  InitialCondition=ess_module_num*mean(ess_voc(1,:))
  MinMax : MinMax  Inputs=2  InputSameDT=on  SaturateOnIntegerOverflow=on
  Product1 : Product  InputSameDT=on  RndMeth=Zero  SaturateOnIntegerOverflow=on  OutDataTypeStr=Inherit: Same as first input
  Relational Operator : RelationalOperator  Operator=<=  RndMeth=Nearest  InputSameDT=on
  Relational Operator2 : RelationalOperator  Operator===  RndMeth=Nearest  InputSameDT=on
  Sign : Subsystem  mask(Sign){}
      mask help: y = sign(x)
      mask Help: Sign Function:\n\t\t\ty = 1 if x > 0\n\t\t\ty = 0 if x = 0\n\t\t\ty = -1 if x < 0
      mask Display: plot(-50,-50,50,50,[-50,50],[0,0],[0,0],[-50,50],[-40,0],[-30,-30],[0,40],[30,30])
  Switch : Switch  Threshold=eps  SaturateOnIntegerOverflow=on  InputSameDT=on
  current-limited power : Product  InputSameDT=on  RndMeth=Zero  SaturateOnIntegerOverflow=on  OutDataTypeStr=Inherit: Same as first input
  true if motor should be shut down : Logic  Operator=OR
  req'd input power (W)1 : Outport  InitialOutput=0
  tag scope: mc_crrnt_limited=global
  wires:
  shifting/1 -> true if motor should be shut down/2
  Logical Operator1/1 -> Switch/2
  true if motor should be shut down/1 -> Logical Operator1/1
  Memory/1 -> Product1/1
  bus voltage/1 -> Memory/1
  Constant/1 -> Product1/2
  req'd input power (W)/1 -> Abs/1, Sign/1(in_1)
  Abs/1 -> MinMax/2
  Sign/1(out_1) -> current-limited power/2
  Constant2/1 -> Switch/3
  Switch/1 -> req'd input power (W)1/1
  current-limited power/1 -> Switch/1
  Product1/1 -> MinMax/1, Relational Operator2/1
  MinMax/1 -> current-limited power/1, Relational Operator2/2
  Relational Operator2/1 -> [mc_crrnt_limited]
  Relational Operator/1 -> true if motor should be shut down/1
  Constant1/1 -> Relational Operator/2
  req'd output spd (rad/s)/1 -> Abs1/1
  Abs1/1 -> Relational Operator/1

== system BD_PAR_SS/<vc> par/parallel clutch control ==
  shifting : Inport
  gb_trq_in_r : Inport  Port=2
  gb_spd_in_r : Inport  Port=3
  engine on : Inport  Port=4
  Block NOTES : Subsystem
      mask Display: disp('Block\nNOTES')
  Clock : Clock
  Constant : Constant  Value=1e-3
  Constant1 : Constant  Value=vc_clutch_bool
  Constant2 : Constant  Value=vc_idle_spd
  Constant3 : Constant  Value=1e-3
  Constant4 : Constant  Value=vc_launch_spd
  Constant5 : Constant  Value=2.5
  Constant6 : Constant
  Fcn: 1 if clutch disengaged 2 if clutch slipping 3 if clutch engaged : Fcn  Expr=u[1]+2*u[2]*(1-u[1])*(1-u[3])+3*u[3]*(1-u[1])
  Logical Operator : Logic
  Logical Operator1 : Logic  Operator=OR
  Manual Switch : ManualSwitch
  Memory : Memory  InitialCondition=1+(2*(cyc_mph(1,2)>0))
  Memory1 : Memory  InitialCondition=cyc_mph(1,2)>0
  Memory2 : Memory  InitialCondition=-1
  Mux : Mux  Inputs=3
  Relational Operator : RelationalOperator  Operator=<=  RndMeth=Nearest  InputSameDT=on
  Relational Operator1 : RelationalOperator  Operator=<  RndMeth=Nearest  InputSameDT=on
  Relational Operator2 : RelationalOperator  Operator=>  RndMeth=Nearest  InputSameDT=on
  Relational Operator3 : RelationalOperator  Operator=<  RndMeth=Nearest  InputSameDT=on
  Sum : Sum  Inputs=+-  InputSameDT=on  SaturateOnIntegerOverflow=on  OutDataTypeStr=Inherit: Same as first input
  Switch : Switch  Threshold=eps  SaturateOnIntegerOverflow=on  InputSameDT=on
  Switch1 : Switch  Threshold=0.5  SaturateOnIntegerOverflow=on  InputSameDT=on
  Transport Delay : TransportDelay
  clutch disengaged : Logic  Operator=OR
  clutch engaged : Logic  Operator=NOR
  clutch slipping : Logic  Inputs=3
  clutch slipping1 : Logic
  clutch slipping2 : Logic
  clutch was NOT fully engaged during last time step : RelationalOperator  Operator=<  RndMeth=Nearest  InputSameDT=on
  gearbox speed estimator : Subsystem
  clutch state : Outport
  wires:
  Switch/1 -> Memory/1, clutch state/1
  Fcn: 1 if clutch disengaged 2 if clutch slipping 3 if clutch engaged/1 -> Switch/1
  Manual Switch/1 -> Switch/2
  Switch1/1 -> Manual Switch/2
  gearbox speed estimator/1(Out1) -> Relational Operator3/1, Relational Operator1/1
  gb_spd_in_r/1 -> gearbox speed estimator/1(gb_spd_in_r if no gear change)
  Sum/1 -> Switch1/2
  Memory2/1 -> Sum/2
  Clock/1 -> Memory2/1, Sum/1
  clutch slipping2/1 -> Switch1/3
  Transport Delay/1 -> clutch slipping2/2
  clutch slipping1/1 -> Switch1/1
  Memory1/1 -> clutch slipping1/2
  engine on/1 -> Manual Switch/1, clutch slipping2/1, Transport Delay/1, Memory1/1, clutch slipping1/1
  Relational Operator1/1 -> Logical Operator1/2
  Constant2/1 -> Relational Operator1/2
  Mux/1 -> Fcn: 1 if clutch disengaged 2 if clutch slipping 3 if clutch engaged/1
  clutch engaged/1 -> Mux/3
  clutch disengaged/1 -> clutch engaged/1, Mux/1
  Constant3/1 -> Relational Operator2/2
  Relational Operator2/1 -> clutch slipping/1
  clutch slipping/1 -> clutch engaged/2, Mux/2
  Constant4/1 -> Relational Operator3/2
  Relational Operator3/1 -> clutch slipping/2
  Memory/1 -> clutch was NOT fully engaged during last time step/1
  Constant5/1 -> clutch was NOT fully engaged during last time step/2
  clutch was NOT fully engaged during last time step/1 -> clutch slipping/3
  Constant1/1 -> Logical Operator1/1
  Constant/1 -> Relational Operator/2
  Relational Operator/1 -> Logical Operator/1
  Logical Operator1/1 -> Logical Operator/2
  gb_trq_in_r/1 -> Relational Operator2/1, Relational Operator/1
  Logical Operator/1 -> clutch disengaged/2
  shifting/1 -> clutch disengaged/1
  Constant6/1 -> Switch/3

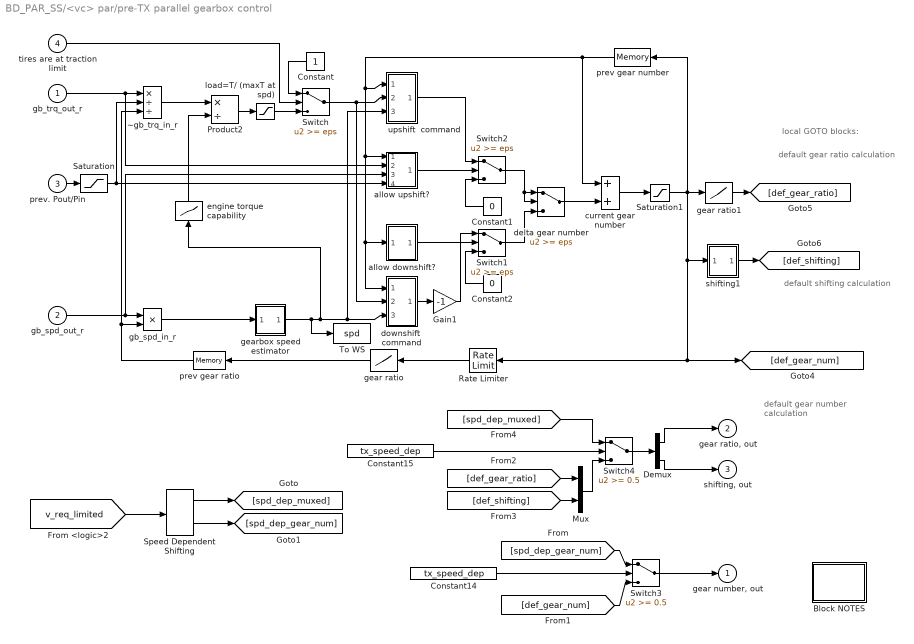
== system BD_PAR_SS/<vc> par/pre-TX parallel gearbox control ==
  note: local GOTO blocks:
  note: default gear ratio
      | calculation
  note: default shifting
      | calculation
  note: default gear number
      | calculation
  gb_trq_out_r : Inport
  gb_spd_out_r : Inport  Port=2
  prev. Pout/Pin : Inport  Port=3
  tires are at traction limit : Inport  Port=4
  Block NOTES : Subsystem
      mask Display: disp('Block\nNOTES')
  Constant : Constant
  Constant1 : Constant  Value=0
  Constant14 : Constant  Value=tx_speed_dep
  Constant15 : Constant  Value=tx_speed_dep
  Constant2 : Constant  Value=0
  Demux : Demux  Outputs=2
      settings: DisplayOption=none
  Gain1 : Gain  Gain=-1  SaturateOnIntegerOverflow=on  OutDataTypeStr=Inherit: Same as input  ParamDataTypeStr=Inherit: Same as input
  Mux : Mux  Inputs=2
  Product2 : Product  Inputs=*/  InputSameDT=on  RndMeth=Zero  SaturateOnIntegerOverflow=on  OutDataTypeStr=Inherit: Same as first input
  Rate Limiter : RateLimiter  RisingSlewLimit=1/(gb_shift_delay+eps)  FallingSlewLimit=-1/(gb_shift_delay+eps)
  Saturation : Saturate  UpperLimit=1  LowerLimit=0.2
  Saturation1 : Saturate  UpperLimit=gb_gears_num  LowerLimit=1
  Speed Dependent Shifting : lib_controls/SubSystem/Speed Dependent Shifting  SystemSampleTime=-1  VariantActivationTime=update diagram  Latency=0  AutoFrameSizeCalculation=off
  Switch : Switch  Threshold=eps  SaturateOnIntegerOverflow=on  InputSameDT=on
  Switch1 : Switch  Threshold=eps  SaturateOnIntegerOverflow=on  InputSameDT=on
  Switch2 : Switch  Threshold=eps  SaturateOnIntegerOverflow=on  InputSameDT=on
  Switch3 : Switch  Threshold=0.5  SaturateOnIntegerOverflow=on  InputSameDT=on
  Switch4 : Switch  Threshold=0.5  SaturateOnIntegerOverflow=on  InputSameDT=on
  To WS : ToWorkspace  VariableName=spd  SampleTime=-1
  allow downshift? : Subsystem
  allow upshift? : Subsystem
  current gear number : Sum  InputSameDT=on  SaturateOnIntegerOverflow=on  OutDataTypeStr=Inherit: Same as first input
  delta gear number : Switch  Threshold=eps  SaturateOnIntegerOverflow=on  InputSameDT=on
  downshift  command : Subsystem
  engine torque capability : Lookup  InputValues=fc_map_spd*fc_spd_scale  Table=fc_max_trq*fc_trq_scale+eps  SaturateOnIntegerOverflow=on
  gb_spd_in_r : Product  InputSameDT=on  RndMeth=Zero  SaturateOnIntegerOverflow=on  OutDataTypeStr=Inherit: Same as first input
  gear ratio : Lookup  InputValues=[1:length(gb_ratio)]  Table=gb_ratio  SaturateOnIntegerOverflow=on
  gear ratio1 : Lookup  InputValues=[1:length(gb_ratio)]  Table=gb_ratio  SaturateOnIntegerOverflow=on
  gearbox speed estimator : Subsystem
  load=T/ (maxT at spd) : Saturate  UpperLimit=1  LowerLimit=0
  prev gear number : Memory  InitialCondition=gb_num_init
  prev gear ratio : Memory  InitialCondition=gb_ratio(gb_num_init)
  shifting1 : Subsystem
  upshift  command : Subsystem
  ~gb_trq_in_r : Product  Inputs=*//  InputSameDT=on  RndMeth=Zero  SaturateOnIntegerOverflow=on  OutDataTypeStr=Inherit: Same as first input
  "gear number, out" : Outport  InitialOutput=0
  "gear ratio, out" : Outport  Port=2  InitialOutput=0
  "shifting, out" : Outport  Port=3  InitialOutput=0
  wires:
  Switch3/1 -> "gear number, out"/1
  Demux/2 -> "shifting, out"/1
  Demux/1 -> "gear ratio, out"/1
  Speed Dependent Shifting/2 -> [spd_dep_gear_num]
  Speed Dependent Shifting/1 -> [spd_dep_muxed]
  [v_req_limited] -> Speed Dependent Shifting/1
  [spd_dep_gear_num] -> Switch3/1
  Switch4/1 -> Demux/1
  [def_shifting] -> Mux/2
  [def_gear_ratio] -> Mux/1
  Mux/1 -> Switch4/3
  [spd_dep_muxed] -> Switch4/1
  Constant15/1 -> Switch4/2
  [def_gear_num] -> Switch3/3
  Constant14/1 -> Switch3/2
  gearbox speed estimator/1(Out1) -> To WS/1, downshift  command/3(engine speed), upshift  command/3(engine speed), engine torque capability/1
  allow upshift?/1(allow shift) -> Switch2/2
  upshift  command/1(command) -> Switch2/1
  Switch/1 -> downshift  command/2(engine load), upshift  command/2(engine load)
  Constant/1 -> Switch/1
  tires are at traction limit/1 -> Switch/2
  ~gb_trq_in_r/1 -> Product2/1
  Product2/1 -> load=T/ (maxT at spd)/1
  Rate Limiter/1 -> gear ratio/1
  gear ratio/1 -> prev gear ratio/1
  prev gear ratio/1 -> gb_spd_in_r/2, ~gb_trq_in_r/3
  gb_trq_out_r/1 -> ~gb_trq_in_r/1, allow upshift?/2(gb_trq_out_r)
  gb_spd_out_r/1 -> gb_spd_in_r/1, allow upshift?/3(gb_spd_out_r)
  Gain1/1 -> Switch1/1
  Constant2/1 -> Switch1/3
  Saturation/1 -> ~gb_trq_in_r/2, allow upshift?/4(prev Pout/Pin)
  prev. Pout/Pin/1 -> Saturation/1
  Constant1/1 -> Switch2/3
  prev gear number/1 -> current gear number/1, upshift  command/1(prev gear number), downshift  command/1(prev gear number), allow upshift?/1(prev gearnum), allow downshift?/1(prev gearnum)
  gear ratio1/1 -> [def_gear_ratio]
  Saturation1/1 -> [def_gear_num], Rate Limiter/1, shifting1/1(gear number), gear ratio1/1, prev gear number/1
  current gear number/1 -> Saturation1/1
  delta gear number/1 -> current gear number/2
  shifting1/1(out_1) -> [def_shifting]
  Switch2/1 -> delta gear number/1, delta gear number/2
  Switch1/1 -> delta gear number/3
  engine torque capability/1 -> Product2/2
  downshift  command/1(command) -> Gain1/1
  allow downshift?/1(allow shift) -> Switch1/2
  load=T/ (maxT at spd)/1 -> Switch/3
  gb_spd_in_r/1 -> gearbox speed estimator/1(gb_spd_in_r if no gear change)
